simulink model "QuarterCarModel_uMR"  (R2019b)
settings: Solver=FixedStepAuto  StartTime=0.0  StopTime=t_tot  FixedStep=dt  RelTol=1e-3
values from neighbouring files (symbols this model uses):
  c_min = 800    [QuarterCarModel.m]
  er = 0.7    [QuarterCarModel.m]
  k = 27000    [QuarterCarModel.m]
  k0 = 38000    [QuarterCarModel.m]
  kt = 300000    [QuarterCarModel.m]
  ms = 450    [QuarterCarModel.m]
  mu = 70    [QuarterCarModel.m]
  wr = 2*pi*v/lc    (= 7.85398163397)    [QuarterCarModel.m]
undefined symbols (not defined in the file or in its folder): val_uMR
libraries: simulink x1
settings Model: Creator=Elia  LastModifiedBy=Elia

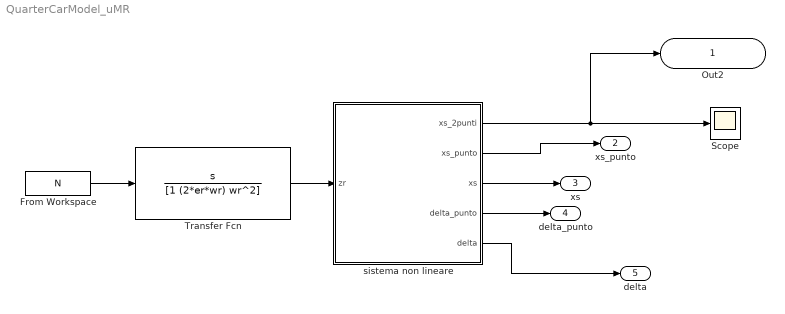
== system QuarterCarModel_uMR ==
  From Workspace : FromWorkspace  VariableName=N  SampleTime=0
  Scope : Scope
  Transfer Fcn : TransferFcn  Numerator=[1 0]  Denominator=[1 (2*er*wr) wr^2]
  sistema non lineare : Subsystem
  Out2 : Outport  SignalName=xs_2punti
  xs_punto : Outport  Port=2  SignalName=xs_punto
  xs : Outport  Port=3  SignalName=xs
  delta_punto : Outport  Port=4  SignalName=delta_punto
  delta : Outport  Port=5  SignalName=delta
  wires:
  From Workspace/1 -> Transfer Fcn/1
  sistema non lineare/1(xs_2punti) -> Scope/1, Out2/1
  Transfer Fcn/1 -> sistema non lineare/1(zr)
  sistema non lineare/2(xs_punto) -> xs_punto/1
  sistema non lineare/3(xs) -> xs/1
  sistema non lineare/4(delta_punto) -> delta_punto/1
  sistema non lineare/5(delta) -> delta/1

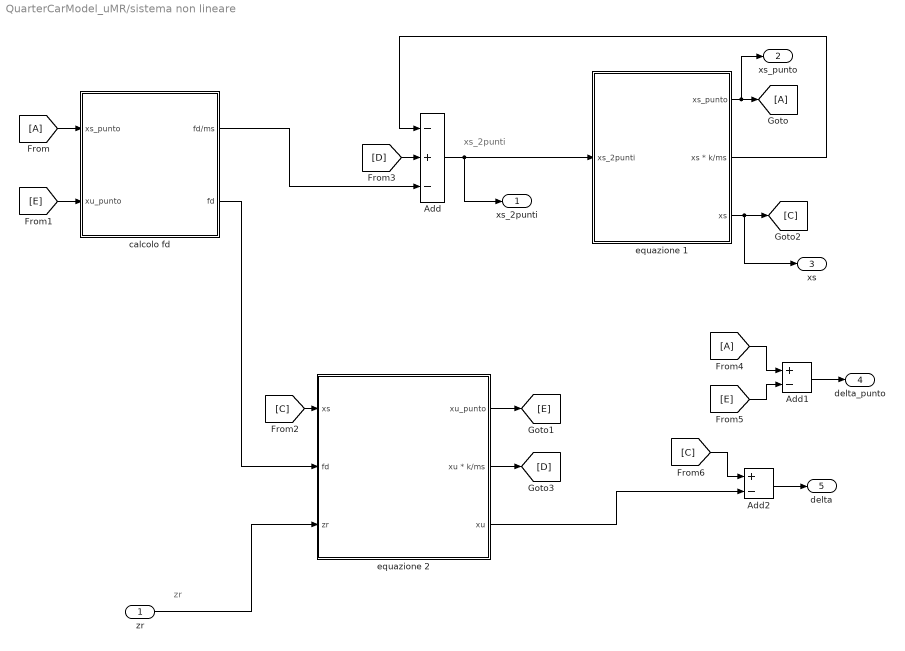
== system QuarterCarModel_uMR/sistema non lineare ==
  note: xs_2punti
  note: zr
  zr : Inport
  Add : Sum  Inputs=-+-
  Add1 : Sum  Inputs=+-
  Add2 : Sum  Inputs=+-
  calcolo fd : Subsystem
  equazione 1 : Subsystem
  equazione 2 : Subsystem
  xs_2punti : Outport
  xs_punto : Outport  Port=2
  xs : Outport  Port=3
  delta_punto : Outport  Port=4
  delta : Outport  Port=5
  wires:
  calcolo fd/2(fd) -> equazione 2/2(fd)
  equazione 1/3(xs) -> xs/1, [C]
  Add/1 -> xs_2punti/1, equazione 1/1(xs_2punti)
  equazione 1/1(xs_punto) -> xs_punto/1, [A]
  calcolo fd/1(fd/ms) -> Add/3
  [C] -> equazione 2/1(xs)
  [D] -> Add/2
  equazione 1/2("xs * k/ms ") -> Add/1
  equazione 2/2("xu * k/ms ") -> [D]
  [A] -> calcolo fd/1(xs_punto)
  zr/1 -> equazione 2/3(zr)
  equazione 2/1(xu_punto) -> [E]
  [E] -> calcolo fd/2(xu_punto)
  [E] -> Add1/2
  [A] -> Add1/1
  Add1/1 -> delta_punto/1
  [C] -> Add2/1
  equazione 2/3(xu) -> Add2/2
  Add2/1 -> delta/1

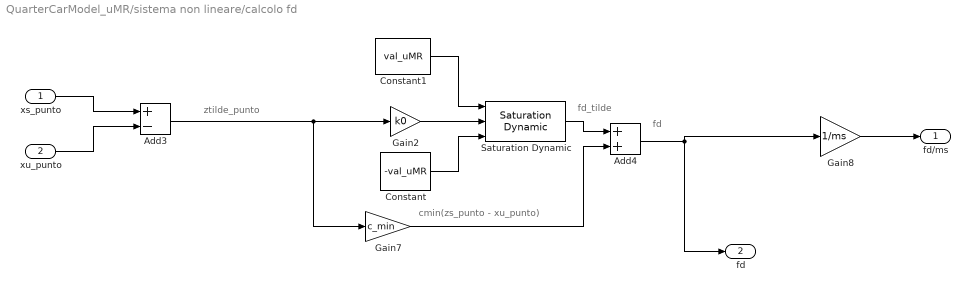
== system QuarterCarModel_uMR/sistema non lineare/calcolo fd ==
  note: ztilde_punto
  note: cmin(zs_punto - xu_punto)
  note: fd
  note: fd_tilde
  xs_punto : Inport
  xu_punto : Inport  Port=2
  Add3 : Sum  Inputs=+-
  Add4 : Sum
  Constant : Constant  Value=-val_uMR
  Constant1 : Constant  Value=val_uMR
  Gain2 : Gain  Gain=k0
  Gain7 : Gain  Gain=c_min
  Gain8 : Gain  Gain=1/ms
  Saturation Dynamic : simulink/Discontinuities/Saturation Dynamic  OutMin=[]  OutMax=[]  OutDataTypeStr=Inherit: Same as second input  OutDataType=fixdt(1, 16)  OutScaling=2^-10  DoSatur=off
  fd/ms : Outport
  fd : Outport  Port=2
  wires:
  Add3/1 -> Gain2/1, Gain7/1
  Gain2/1 -> Saturation Dynamic/2
  xu_punto/1 -> Add3/2
  Add4/1 -> Gain8/1, fd/1
  Gain8/1 -> fd/ms/1
  Gain7/1 -> Add4/2
  Saturation Dynamic/1 -> Add4/1
  Constant1/1 -> Saturation Dynamic/1
  xs_punto/1 -> Add3/1
  Constant/1 -> Saturation Dynamic/3

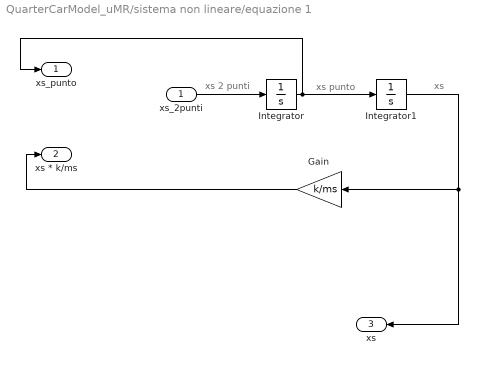
== system QuarterCarModel_uMR/sistema non lineare/equazione 1 ==
  note: xs
  note: xs 2 punti
  note: xs punto
  xs_2punti : Inport
  Gain : Gain  Gain=k/ms
  Integrator : Integrator
  Integrator1 : Integrator
  xs_punto : Outport
  "xs * k/ms " : Outport  Port=2
  xs : Outport  Port=3
  wires:
  xs_2punti/1 -> Integrator/1
  Integrator/1 -> xs_punto/1, Integrator1/1
  Integrator1/1 -> xs/1, Gain/1
  Gain/1 -> "xs * k/ms "/1

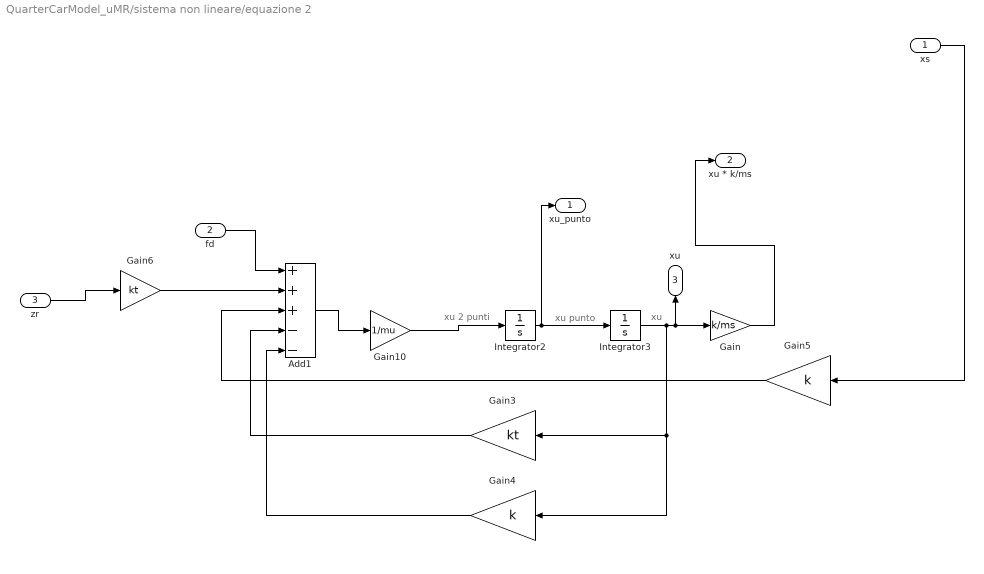
== system QuarterCarModel_uMR/sistema non lineare/equazione 2 ==
  note: xu
  note: xu 2 punti
  note: xu punto
  xs : Inport
  fd : Inport  Port=2
  zr : Inport  Port=3
  Add1 : Sum  Inputs=+++--
  Gain : Gain  Gain=k/ms
  Gain10 : Gain  Gain=1/mu
  Gain3 : Gain  Gain=kt
  Gain4 : Gain  Gain=k
  Gain5 : Gain  Gain=k
  Gain6 : Gain  Gain=kt
  Integrator2 : Integrator
  Integrator3 : Integrator
  xu_punto : Outport
  "xu * k/ms " : Outport  Port=2
  xu : Outport  Port=3
  wires:
  Integrator2/1 -> xu_punto/1, Integrator3/1
  Integrator3/1 -> Gain3/1, Gain4/1, xu/1, Gain/1
  Gain6/1 -> Add1/2
  Add1/1 -> Gain10/1
  Gain10/1 -> Integrator2/1
  Gain3/1 -> Add1/4
  Gain5/1 -> Add1/3
  Gain4/1 -> Add1/5
  zr/1 -> Gain6/1
  xs/1 -> Gain5/1
  fd/1 -> Add1/1
  Gain/1 -> "xu * k/ms "/1
